simulink model "doppiopendolo"  (R2020b)
settings: Solver=ode23  StartTime=0.0  StopTime=10  RelTol=1e-3
settings Model: Creator=Lenovo  LastModifiedBy=Lenovo
settings SolverCC: ShapePreserveControl=EnableAll

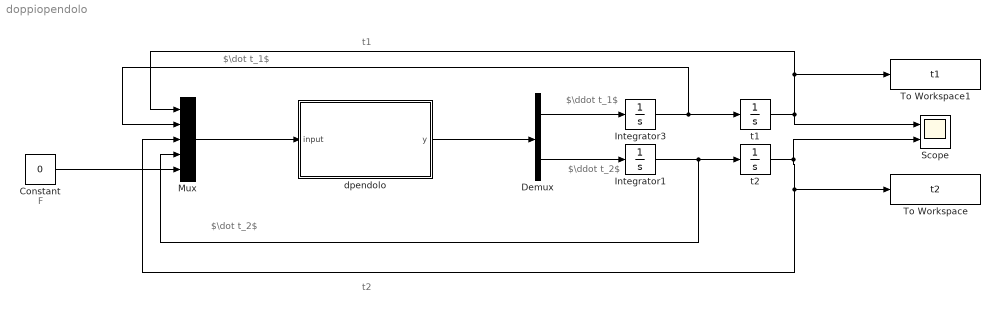
== system doppiopendolo ==
  note: t2
  note: t1
  note: $\dot t_2$
  note: $\dot t_1$
  note: F
  note: $\ddot t_1$
  note: $\ddot t_2$
  Constant : Constant  Value=0
  Demux : Demux  Outputs=2
  Integrator1 : Integrator
  Integrator3 : Integrator
  Mux : Mux  Inputs=5
  Scope : Scope  NumInputPorts=2
  To Workspace : ToWorkspace  VariableName=t2  SampleTime=-1
  To Workspace1 : ToWorkspace  VariableName=t1  SampleTime=-1
  dpendolo : MATLAB Function  TreatAsAtomicUnit=on
  t1 : Integrator  InitialCondition=pi/4
  t2 : Integrator
  wires:
  dpendolo/1(y) -> Demux/1
  Demux/1 -> Integrator3/1
  Integrator3/1 -> Mux/2, t1/1
  Integrator1/1 -> Mux/4, t2/1
  Demux/2 -> Integrator1/1
  Mux/1 -> dpendolo/1(input)
  t1/1 -> To Workspace1/1, Mux/1, Scope/1
  t2/1 -> Mux/3, To Workspace/1, Scope/2
  Constant/1 -> Mux/5

== matlab function doppiopendolo/dpendolo ==
  data: input input; y output
function y = dpendolo(input)

m1 = 0.5;
m2 = 0.5;
L1 = 1;
L2 = 1;
g=9.81;
y=[0;0];

t1=input(1);
dt1=input(2);
t2 = input (3);
dt2= input (4);
F = input (5);

A = [(m1+m2)*(L1^2), m2*L1*L2*cos(t2-t1);m2*L1*L2*cos(t2-t1), m2*L2^2];
B = [F*L1*cos(t1)+m2*L1*L2*(dt2^2)*sin(t2-t1)-(m1+m2)*g*L1*sin(t1);-m2*L1*L2*dt1^2*sin(t2-t1)+F*L2*cos(t2)-m2*g*L2*sin(t2)];

y = inv(A)*B;
